simulink model "model"  (R2021a)
settings: Solver=ode45  StartTime=0.0  StopTime=2400  MaxStep=0.1  RelTol=1e-3
values from neighbouring files (symbols this model uses):
  fc_fuel_map_gpkWh = fc_fuel_map./fc_map_kW*3600    [FC_SI95.m]    (also in FC_SI95.mat = [612 612 612 594 558 522 468 522 540 684 756 756 ... (132 el)
  fc_map_spd = [0.5:0.5:6]*1000*2*pi/60    [FC_SI95.m]    (also in FC_SI95.mat = [52.3598775598 104.71975512 157.079632679 209.439510239 261.)
  fc_map_trq = [1:11]*15.6    [FC_SI95.m]    (also in FC_SI95.mat = [15.6 31.2 46.8 62.4 78 93.6 109.2 124.8 140.4 156 171.6])
  mc_eff_map = [0.78 0.79 0.8 0.811 0.811 0.817 0.82 0.828 0.837 0.845 0.862 0.876 ... (1125 elements, 45x25)]    [PM_UQM_motor_100kW.mat]
  mc_map_spd = [0 10.471975512 20.9439510239 31.4159265359 41.8879020479 52.3598775598 62.8318530718 73.3038285838 83.7758040957 94.2477796077 104.71975512 115.191730632 ... (45 elements, 1x45)]    [PM_UQM_motor_100kW.mat]
  mc_map_trq = [-600 -550 -500 -450 -400 -350 -300 -250 -200 -150 -100 -50 ... (25 elements, 1x25)]    [PM_UQM_motor_100kW.mat]
settings Model: Creator=Wlodzimierz  LastModifiedBy=48508
settings SolverCC: ZeroCrossAlgorithm=Adaptive  AlgebraicLoopSolver=TrustRegion
settings DebuggingCC: IgnoredZcDiagnostic=none  SFMachineParentedDataDiag=warning

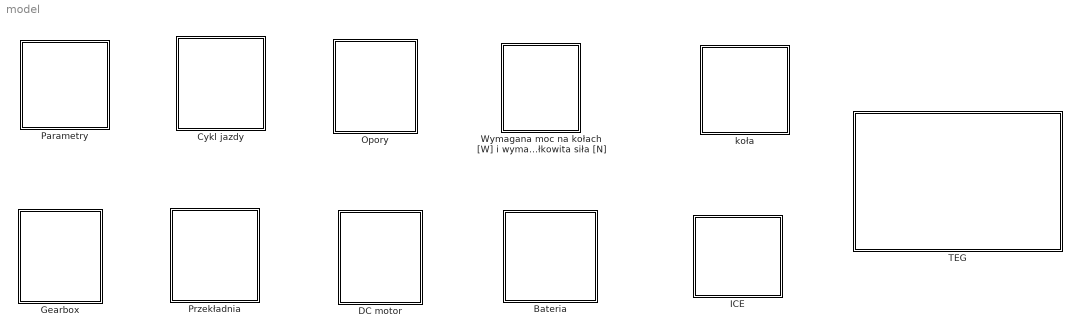
== system model ==
  Bateria : Subsystem
  Cykl jazdy : Subsystem
  DC motor : Subsystem
  Gearbox : Subsystem
  ICE : Subsystem
  Opory : Subsystem
  Parametry : Subsystem  mask{m1_=1500, f1_=0.001, cx_=0.27, a_=2.01, rd_=0.32, prz_=3.46, eta_kwm_=0.95}
      mask prompts: m1_ "masa"; f1_ "wsp. op. tocz."; cx_ "wsp. op. aerodynamicznych cx"; a_ "pow. czołowa [m^2]"; rd_ "promień koła [m]"; prz_ "przełożenie silnik-koła"; eta_kwm_ "sprawność przekładni"
  Przekładnia : Subsystem
  TEG : Subsystem
  Wymagana moc na kołach [W] i wymagana całkowita siła [N] : Subsystem
  koła : Subsystem

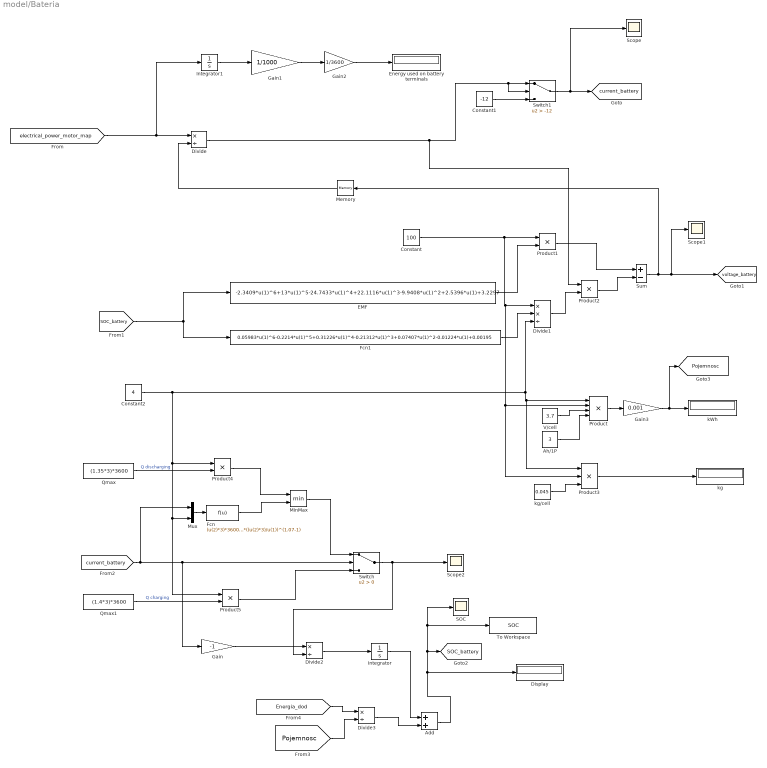
== system model/Bateria ==
  Add : Sum
  Ah/1P : Constant  Value=3
  Constant : Constant  Value=100
  Constant1 : Constant  Value=-12
  Constant2 : Constant  Value=4
  Display : Display
  Divide : Product  Inputs=*/
  Divide1 : Product  Inputs=**/
  Divide2 : Product  Inputs=*/
  Divide3 : Product  Inputs=*/
  EMF : Fcn  Expr=-2.3409*u(1)^6+13*u(1)^5-24.7433*u(1)^4+22.1116*u(1)^3-9.9408*u(1)^2+2.5396*u(1)+3.2297
  Energy used on battery terminals : Display
  Fcn : Fcn  Expr=(u(2)*3)*3600*((u(2)*3)/u(1))^(1.07-1)
  Fcn1 : Fcn  Expr=0.05983*u(1)^6-0.2214*u(1)^5+0.31226*u(1)^4-0.21312*u(1)^3+0.07407*u(1)^2-0.01224*u(1)+0.00195
  Gain : Gain  Gain=-1
  Gain1 : Gain  Gain=1/1000
  Gain2 : Gain  Gain=1/3600
  Gain3 : Gain  Gain=0.001
  Integrator : Integrator  InitialCondition=0.65
  Integrator1 : Integrator
  Memory : Memory  InitialCondition=500
  MinMax : MinMax  Inputs=2  ZeroCross=off
  Mux : Mux  Inputs=2
  Product : Product  Inputs=4
  Product{1..2,4..5} (4 alike) : Product
  Product3 : Product  Inputs=3
  Qmax : Constant  Value=(1.35*3)*3600
  Qmax1 : Constant  Value=(1.4*3)*3600
  SOC : Scope
  Scope : Scope
  Scope1 : Scope
  Scope2 : Scope
  Sum : Sum  Inputs=+-
  Switch : Switch  Criteria=u2 > Threshold  ZeroCross=off
  Switch1 : Switch  Criteria=u2 > Threshold  Threshold=-12
  To Workspace : ToWorkspace  VariableName=SOC  SaveFormat=Timeseries  SampleTime=-1
  V/cell : Constant  Value=3.7
  kWh : Display
  kg : Display
  kg/cell : Constant  Value=0.045
  tag scope: Pojemnosc=global, SOC_battery=global, current_battery=global, voltage_battery=global
  wires:
  Divide/1 -> Product2/1, Switch1/2, Switch1/1
  [SOC_battery] -> EMF/1, Fcn1/1
  Fcn1/1 -> Divide1/2
  Constant2/1 -> Mux/2, Product5/1, Product4/1, Divide1/3, Product3/1, Product/1
  Divide1/1 -> Product2/2
  Product2/1 -> Sum/2
  Sum/1 -> Memory/1, Scope1/1, [voltage_battery]
  EMF/1 -> Product1/2
  Product1/1 -> Sum/1
  Constant/1 -> Product3/2, Product/2, Divide1/1, Product1/1
  Memory/1 -> Divide/2
  Ah/1P/1 -> Product/4
  V/cell/1 -> Product/3
  kg/cell/1 -> Product3/3
  Product3/1 -> kg/1
  Product/1 -> Gain3/1
  Gain/1 -> Divide2/1
  Fcn/1 -> MinMax/2
  MinMax/1 -> Switch/1
  Divide2/1 -> Integrator/1
  Switch/1 -> Scope2/1, Divide2/2
  [current_battery] -> Mux/1, Gain/1, Switch/2
  Qmax/1 -> Product4/2  "Q discharging"
  Mux/1 -> Fcn/1
  Product4/1 -> MinMax/1
  Qmax1/1 -> Product5/2  "Q charging"
  Product5/1 -> Switch/3
  Integrator1/1 -> Gain1/1
  Gain1/1 -> Gain2/1
  Gain2/1 -> Energy used on battery terminals/1
  [electrical_power_motor_map] -> Divide/1, Integrator1/1
  Gain3/1 -> [Pojemnosc], kWh/1
  Constant1/1 -> Switch1/3
  Switch1/1 -> Scope/1, [current_battery]
  [Pojemnosc] -> Divide3/2
  [Energia_dod] -> Divide3/1
  Divide3/1 -> Add/2
  Integrator/1 -> Add/1
  Add/1 -> Display/1, To Workspace/1, SOC/1, [SOC_battery]

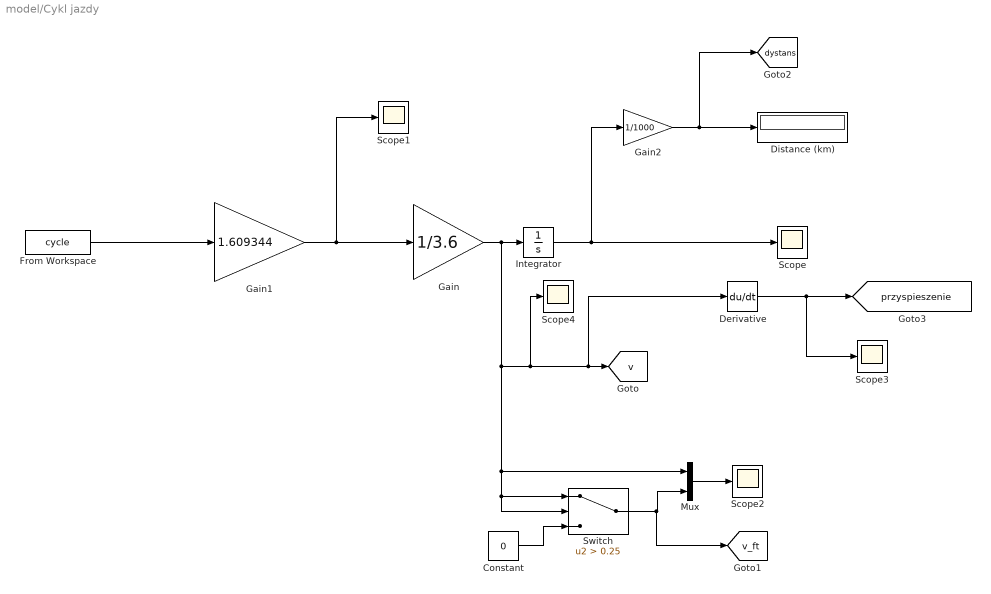
== system model/Cykl jazdy ==
  Constant : Constant  Value=0
  Derivative : Derivative
  Distance (km) : Display
  From Workspace : FromWorkspace  VariableName=cycle
  Gain : Gain  Gain=1/3.6
  Gain1 : Gain  Gain=1.609344
  Gain2 : Gain  Gain=1/1000
  Integrator : Integrator
  Mux : Mux  Inputs=2
  Scope{,1..4} (5 alike) : Scope
  Switch : Switch  Criteria=u2 > Threshold  Threshold=0.25
  tag scope: dystans=global, przyspieszenie=global, v=global, v_ft=global
  wires:
  Mux/1 -> Scope2/1
  Integrator/1 -> Scope/1, Gain2/1
  Gain1/1 -> Gain/1, Scope1/1
  Gain/1 -> Mux/1, Switch/2, Switch/1, Scope4/1, Derivative/1, [v], Integrator/1
  Switch/1 -> [v_ft], Mux/2
  Constant/1 -> Switch/3
  Gain2/1 -> [dystans], Distance (km)/1
  Derivative/1 -> Scope3/1, [przyspieszenie]
  From Workspace/1 -> Gain1/1

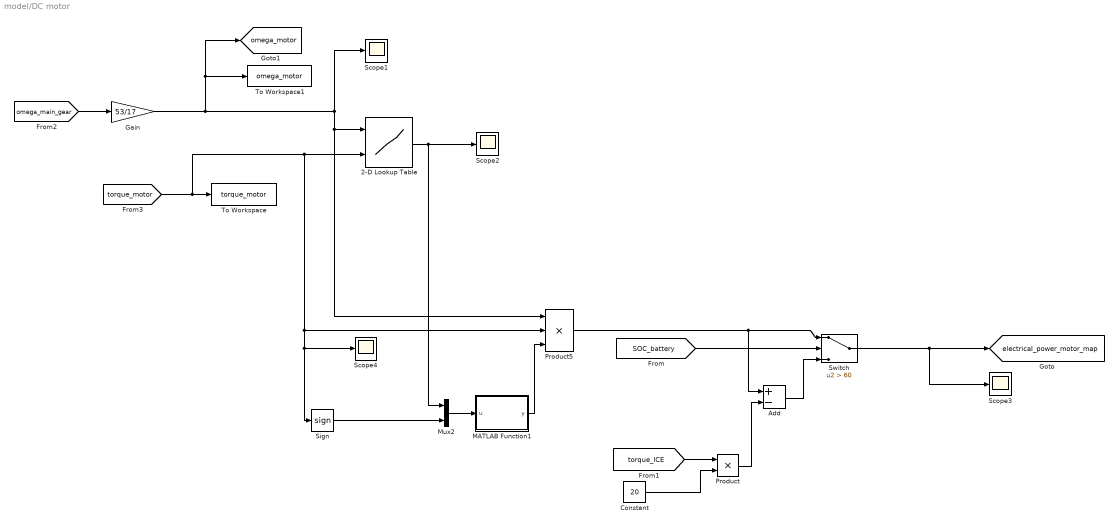
== system model/DC motor ==
  2-D Lookup Table : Lookup_n-D  BreakpointsForDimension1=mc_map_spd*3  BreakpointsForDimension2=mc_map_trq*0.2  Table=mc_eff_map  InternalRulePriority=Speed  RndMeth=Simplest  InputSameDT=on
      settings: InputPortMap=u0,u1
  Add : Sum  Inputs=+-
  Constant : Constant  Value=20
  Gain : Gain  Gain=53/17
  MATLAB Function1 : MATLAB Function  TreatAsAtomicUnit=on
  Mux2 : Mux  Inputs=2
  Product : Product
  Product5 : Product  Inputs=3
  Scope{1..4} (4 alike) : Scope
  Sign : Signum
  Switch : Switch  Criteria=u2 > Threshold  Threshold=60
  To Workspace : ToWorkspace  VariableName=torque_motor  SampleTime=1
  To Workspace1 : ToWorkspace  VariableName=omega_motor  SampleTime=1
  tag scope: electrical_power_motor_map=global, omega_motor=global
  wires:
  Sign/1 -> Mux2/2
  2-D Lookup Table/1 -> Mux2/1, Scope2/1
  Mux2/1 -> MATLAB Function1/1(u)
  MATLAB Function1/1(y) -> Product5/3
  [torque_motor] -> Scope4/1, Sign/1, Product5/2, 2-D Lookup Table/2, To Workspace/1
  [omega_main_gear] -> Gain/1
  [torque_ICE] -> Product/1
  Constant/1 -> Product/2
  [SOC_battery] -> Switch/2
  Product5/1 -> Add/1, Switch/1
  Product/1 -> Add/2
  Add/1 -> Switch/3
  Switch/1 -> Scope3/1, [electrical_power_motor_map]
  Gain/1 -> [omega_motor], To Workspace1/1, Product5/1, 2-D Lookup Table/1, Scope1/1

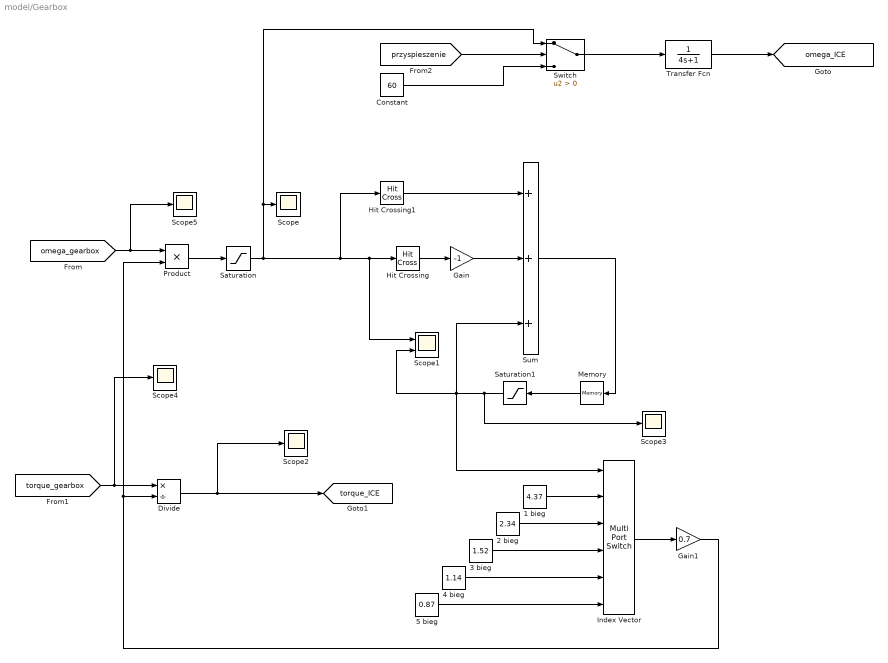
== system model/Gearbox ==
  1 bieg : Constant  Value=4.37
  2 bieg : Constant  Value=2.34
  3 bieg : Constant  Value=1.52
  4 bieg : Constant  Value=1.14
  5 bieg : Constant  Value=0.87
  Constant : Constant  Value=60
  Divide : Product  Inputs=*/
  Gain : Gain  Gain=-1
  Gain1 : Gain  Gain=0.7
  Hit Crossing : HitCross  HitCrossingOffset=120  HitCrossingDirection=falling
  Hit Crossing1 : HitCross  HitCrossingOffset=270  HitCrossingDirection=rising
  Index Vector : MultiPortSwitch  Inputs=5
  Memory : Memory  InitialCondition=1
  Product : Product
  Saturation : Saturate  UpperLimit=280  LowerLimit=80
  Saturation1 : Saturate  UpperLimit=5  LowerLimit=1
  Scope{,2..5} (5 alike) : Scope
  Scope1 : Scope  NumInputPorts=2
  Sum : Sum  Inputs=+++
  Switch : Switch  Criteria=u2 > Threshold
  Transfer Fcn : TransferFcn  Denominator=[4 1]
  tag scope: omega_ICE=global, torque_ICE=global
  wires:
  [omega_gearbox] -> Scope5/1, Product/1
  Product/1 -> Saturation/1
  Saturation/1 -> Switch/1, Scope/1, Scope1/1, Hit Crossing/1, Hit Crossing1/1
  Hit Crossing/1 -> Gain/1
  Hit Crossing1/1 -> Sum/1
  Gain/1 -> Sum/2
  Sum/1 -> Memory/1
  Memory/1 -> Saturation1/1
  Saturation1/1 -> Scope3/1, Index Vector/1, Scope1/2, Sum/3
  [torque_gearbox] -> Scope4/1, Divide/1
  Gain1/1 -> Product/2, Divide/2
  5 bieg/1 -> Index Vector/6
  4 bieg/1 -> Index Vector/5
  3 bieg/1 -> Index Vector/4
  2 bieg/1 -> Index Vector/3
  1 bieg/1 -> Index Vector/2
  Index Vector/1 -> Gain1/1
  Divide/1 -> Scope2/1, [torque_ICE]
  [przyspieszenie] -> Switch/2
  Constant/1 -> Switch/3
  Switch/1 -> Transfer Fcn/1
  Transfer Fcn/1 -> [omega_ICE]

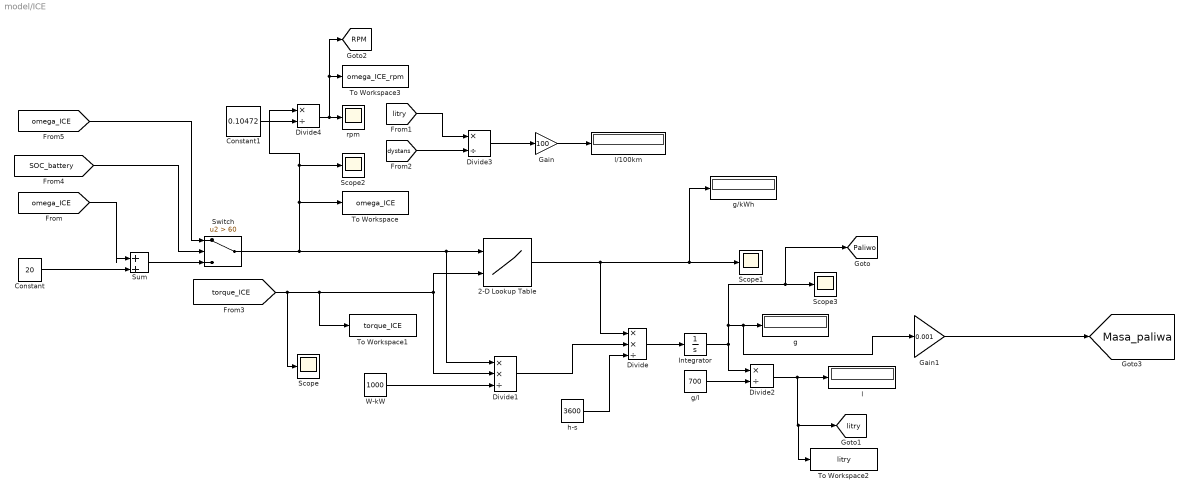
== system model/ICE ==
  2-D Lookup Table : Lookup_n-D  BreakpointsForDimension1=fc_map_spd  BreakpointsForDimension2=fc_map_trq  Table=fc_fuel_map_gpkWh  InternalRulePriority=Speed  RndMeth=Simplest  InputSameDT=on
      settings: InputPortMap=u0,u1
  Constant : Constant  Value=20
  Constant1 : Constant  Value=0.10472
  Divide : Product  Inputs=**/
  Divide1 : Product  Inputs=**/
  Divide2 : Product  Inputs=*/
  Divide3 : Product  Inputs=*/
  Divide4 : Product  Inputs=*/
  Gain : Gain  Gain=100
  Gain1 : Gain  Gain=0.001
  Integrator : Integrator
  Scope{,1..3} (4 alike) : Scope
  Sum : Sum  Inputs=|++
  Switch : Switch  Criteria=u2 > Threshold  Threshold=60
  To Workspace : ToWorkspace  VariableName=omega_ICE  SampleTime=1
  To Workspace1 : ToWorkspace  VariableName=torque_ICE  SampleTime=1
  To Workspace2 : ToWorkspace  VariableName=litry  SaveFormat=Timeseries  SampleTime=-1
  To Workspace3 : ToWorkspace  VariableName=omega_ICE_rpm  SampleTime=1
  W-kW : Constant  Value=1000
  g : Display
  g/kWh : Display
  g/l : Constant  Value=700
  h-s : Constant  Value=3600
  l : Display
  l/100km : Display
  rpm : Scope
  tag scope: Masa_paliwa=global, Paliwo=global, RPM=global, litry=global
  wires:
  W-kW/1 -> Divide1/3
  Divide1/1 -> Divide/2
  Divide/1 -> Integrator/1
  h-s/1 -> Divide/3
  g/l/1 -> Divide2/2
  Integrator/1 -> Gain1/1, g/1, [Paliwo], Scope3/1, Divide2/1
  Divide2/1 -> To Workspace2/1, [litry], l/1
  2-D Lookup Table/1 -> g/kWh/1, Scope1/1, Divide/1
  [dystans] -> Divide3/2
  [litry] -> Divide3/1
  Divide3/1 -> Gain/1
  Gain/1 -> l/100km/1
  [torque_ICE] -> Scope/1, To Workspace1/1, Divide1/2, 2-D Lookup Table/2
  [omega_ICE] -> Sum/1
  Constant/1 -> Sum/2
  [SOC_battery] -> Switch/2
  Sum/1 -> Switch/3
  Switch/1 -> Divide4/1, Scope2/1, To Workspace/1, Divide1/1, 2-D Lookup Table/1
  [omega_ICE] -> Switch/1
  Constant1/1 -> Divide4/2
  Divide4/1 -> [RPM], To Workspace3/1, rpm/1
  Gain1/1 -> [Masa_paliwa]

== system model/Opory ==
  sila oporow bezwladnosci [N] : Subsystem
  sila oporów toczenia [N] : Subsystem
  siła oporów aerodynamicznych [N] : Subsystem

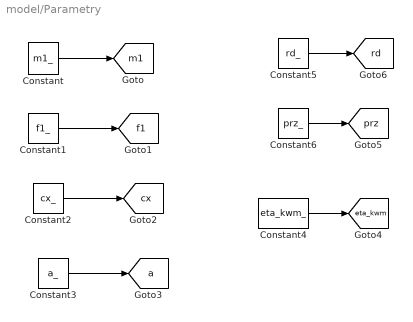
== system model/Parametry ==
  Constant : Constant  Value=m1_
  Constant1 : Constant  Value=f1_
  Constant2 : Constant  Value=cx_
  Constant3 : Constant  Value=a_
  Constant4 : Constant  Value=eta_kwm_
  Constant5 : Constant  Value=rd_
  Constant6 : Constant  Value=prz_
  tag scope: a=global, cx=global, eta_kwm=global, f1=global, m1=global, prz=global, rd=global
  wires:
  Constant1/1 -> [f1]
  Constant/1 -> [m1]
  Constant5/1 -> [rd]
  Constant2/1 -> [cx]
  Constant3/1 -> [a]
  Constant4/1 -> [eta_kwm]
  Constant6/1 -> [prz]

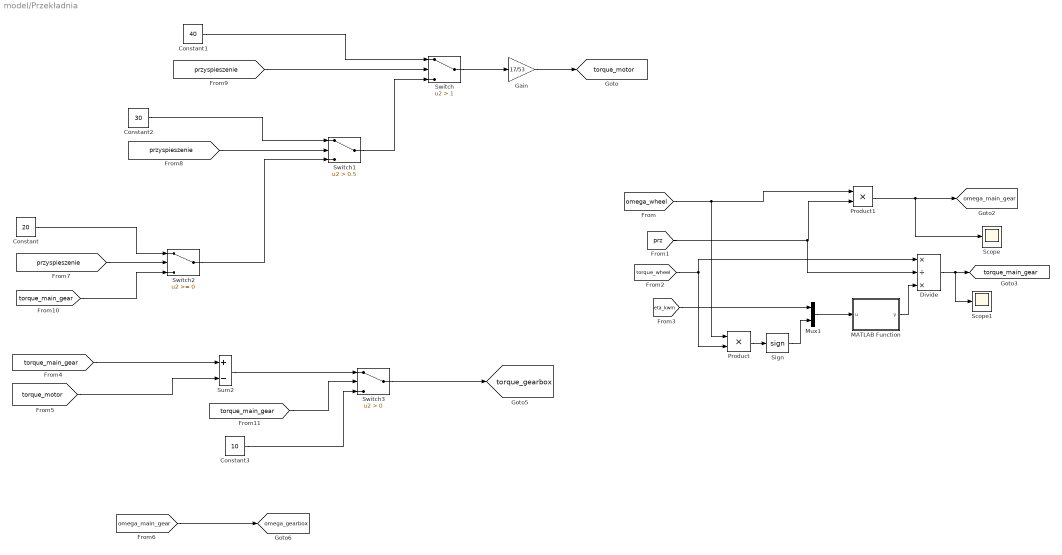
== system model/Przekładnia ==
  Constant : Constant  Value=20
  Constant1 : Constant  Value=40
  Constant2 : Constant  Value=30
  Constant3 : Constant  Value=10
  Divide : Product  Inputs=*/*
  Gain : Gain  Gain=17/53
  MATLAB Function : MATLAB Function  TreatAsAtomicUnit=on
  Mux1 : Mux  Inputs=2
  Product : Product
  Product1 : Product
  Scope : Scope
  Scope1 : Scope
  Sign : Signum
  Sum2 : Sum  Inputs=+-
  Switch : Switch  Criteria=u2 > Threshold  Threshold=1
  Switch1 : Switch  Criteria=u2 > Threshold  Threshold=0.5
  Switch2 : Switch
  Switch3 : Switch  Criteria=u2 > Threshold
  tag scope: omega_gearbox=global, omega_main_gear=global, torque_gearbox=global, torque_main_gear=global, torque_motor=global
  wires:
  MATLAB Function/1(y) -> Divide/3
  Product/1 -> Sign/1
  Divide/1 -> Scope1/1, [torque_main_gear]
  [torque_wheel] -> Product/2, Divide/1
  [eta_kwm] -> Mux1/1
  [omega_wheel] -> Product/1, Product1/1
  Mux1/1 -> MATLAB Function/1(u)
  [prz] -> Divide/2, Product1/2
  Product1/1 -> Scope/1, [omega_main_gear]
  Sign/1 -> Mux1/2
  [torque_main_gear] -> Sum2/1
  [torque_motor] -> Sum2/2
  [przyspieszenie] -> Switch2/2
  [torque_main_gear] -> Switch2/3
  Constant/1 -> Switch2/1
  Switch2/1 -> Switch1/3
  [przyspieszenie] -> Switch1/2
  Switch1/1 -> Switch/3
  [przyspieszenie] -> Switch/2
  Constant2/1 -> Switch1/1
  Constant1/1 -> Switch/1
  Switch/1 -> Gain/1
  Gain/1 -> [torque_motor]
  [omega_main_gear] -> [omega_gearbox]
  Switch3/1 -> [torque_gearbox]
  Sum2/1 -> Switch3/1
  [torque_main_gear] -> Switch3/2
  Constant3/1 -> Switch3/3

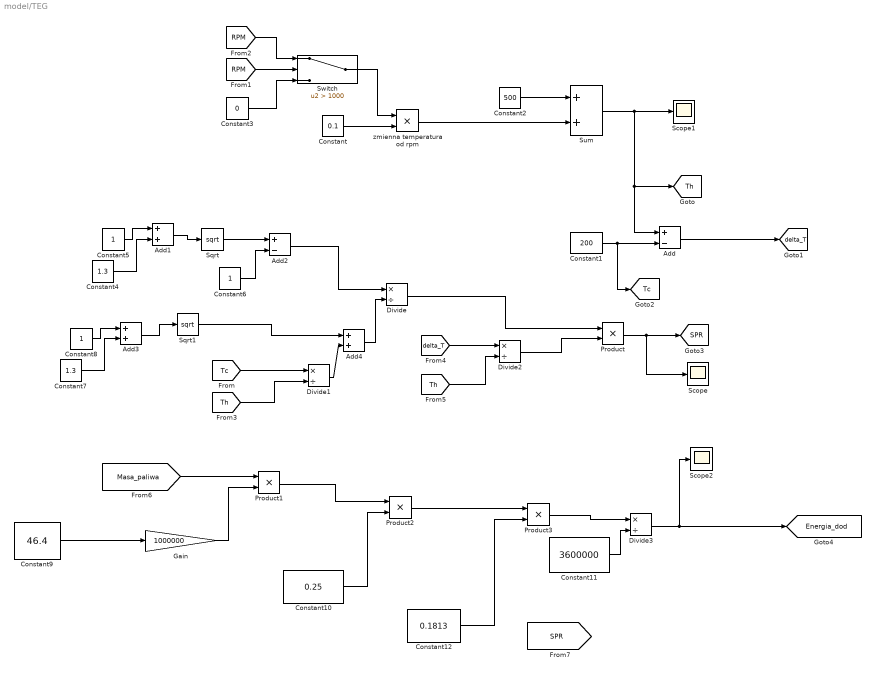
== system model/TEG ==
  Add : Sum  Inputs=+-
  Add1 : Sum
  Add2 : Sum  Inputs=+-
  Add3 : Sum
  Add4 : Sum
  Constant : Constant  Value=0.1
  Constant1 : Constant  Value=200
  Constant10 : Constant  Value=0.25
  Constant11 : Constant  Value=3600000
  Constant12 : Constant  Value=0.1813
  Constant2 : Constant  Value=500
  Constant3 : Constant  Value=0
  Constant4 : Constant  Value=1.3
  Constant5 : Constant
  Constant6 : Constant
  Constant7 : Constant  Value=1.3
  Constant8 : Constant
  Constant9 : Constant  Value=46.4
  Divide{,1..3} (4 alike) : Product  Inputs=*/
  Gain : Gain  Gain=1000000
  Product{,1..3} (4 alike) : Product
  Scope : Scope
  Scope1 : Scope
  Scope2 : Scope
  Sqrt : Sqrt  SaturateOnIntegerOverflow=on
  Sqrt1 : Sqrt  SaturateOnIntegerOverflow=on
  Sum : Sum
  Switch : Switch  Criteria=u2 > Threshold  Threshold=1000
  zmienna temperatura od rpm : Product  Inputs=**
  tag scope: Energia_dod=global, SPR=global, Tc=global, Th=global, delta_T=global
  wires:
  Constant/1 -> zmienna temperatura od rpm/2
  Constant2/1 -> Sum/1
  Sum/1 -> [Th], Add/1, Scope1/1
  zmienna temperatura od rpm/1 -> Sum/2
  [RPM] -> Switch/2
  Constant3/1 -> Switch/3
  Switch/1 -> zmienna temperatura od rpm/1
  [RPM] -> Switch/1
  Constant1/1 -> [Tc], Add/2
  Add/1 -> [delta_T]
  Constant5/1 -> Add1/1
  Constant4/1 -> Add1/2
  Add1/1 -> Sqrt/1
  Sqrt/1 -> Add2/1
  Constant6/1 -> Add2/2
  Add2/1 -> Divide/1
  Constant7/1 -> Add3/2
  Constant8/1 -> Add3/1
  Add3/1 -> Sqrt1/1
  [Tc] -> Divide1/1
  [Th] -> Divide1/2
  Sqrt1/1 -> Add4/1
  Divide1/1 -> Add4/2
  Add4/1 -> Divide/2
  [delta_T] -> Divide2/1
  [Th] -> Divide2/2
  Divide/1 -> Product/1
  Divide2/1 -> Product/2
  Product/1 -> Scope/1, [SPR]
  Constant9/1 -> Gain/1
  Gain/1 -> Product1/2
  [Masa_paliwa] -> Product1/1
  Product1/1 -> Product2/1
  Constant10/1 -> Product2/2
  Product2/1 -> Product3/1
  Product3/1 -> Divide3/1
  Constant11/1 -> Divide3/2
  Divide3/1 -> [Energia_dod], Scope2/1
  Constant12/1 -> Product3/2

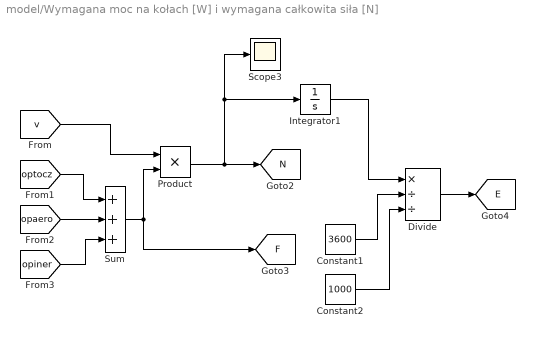
== system model/Wymagana moc na kołach [W] i wymagana całkowita siła [N] ==
  Constant1 : Constant  Value=3600
  Constant2 : Constant  Value=1000
  Divide : Product  Inputs=*//
  Integrator1 : Integrator
  Product : Product
  Scope3 : Scope
  Sum : Sum  Inputs=+++
  tag scope: E=global, F=global, N=global
  wires:
  [opiner] -> Sum/3
  Constant1/1 -> Divide/2
  Constant2/1 -> Divide/3
  [optocz] -> Sum/1
  Divide/1 -> [E]
  [opaero] -> Sum/2
  Product/1 -> Scope3/1, Integrator1/1, [N]
  Integrator1/1 -> Divide/1
  Sum/1 -> Product/2, [F]
  [v] -> Product/1

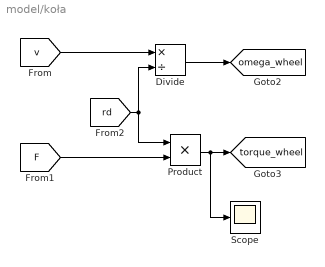
== system model/koła ==
  Divide : Product  Inputs=*/
  Product : Product
  Scope : Scope
  tag scope: omega_wheel=global, torque_wheel=global
  wires:
  [rd] -> Product/1, Divide/2
  Product/1 -> Scope/1, [torque_wheel]
  [F] -> Product/2
  [v] -> Divide/1
  Divide/1 -> [omega_wheel]

== system model/Opory/sila oporow bezwladnosci [N] ==
  Derivative : Derivative
  Product : Product
  Przyspieszenie : Scope
  tag scope: opiner=global
  wires:
  [v] -> Derivative/1
  Derivative/1 -> Przyspieszenie/1, Product/1
  [m1] -> Product/2
  Product/1 -> [opiner]

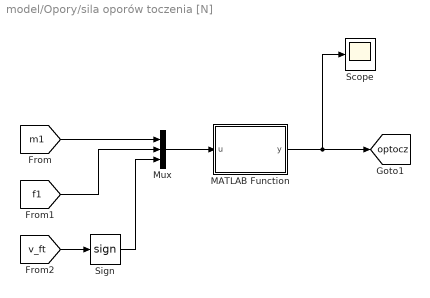
== system model/Opory/sila oporów toczenia [N] ==
  MATLAB Function : MATLAB Function  TreatAsAtomicUnit=on
  Mux : Mux  Inputs=3
  Scope : Scope
  Sign : Signum
  tag scope: optocz=global
  wires:
  [f1] -> Mux/2
  Mux/1 -> MATLAB Function/1(u)
  [m1] -> Mux/1
  [v_ft] -> Sign/1
  Sign/1 -> Mux/3
  MATLAB Function/1(y) -> Scope/1, [optocz]

== system model/Opory/siła oporów aerodynamicznych [N] ==
  MATLAB Function : MATLAB Function  TreatAsAtomicUnit=on
  Mux1 : Mux  Inputs=3
  Scope : Scope
  tag scope: opaero=global
  wires:
  [v] -> Mux1/3
  Mux1/1 -> MATLAB Function/1(u)
  MATLAB Function/1(y) -> Scope/1, [opaero]
  [a] -> Mux1/2
  [cx] -> Mux1/1

== matlab function model/Opory/sila oporów toczenia [N]/MATLAB Function ==
  data: u input; y output
function y = fcn(u)

y = u(1)*9.81*u(2)*u(3);

== matlab function model/Przekładnia/MATLAB Function ==
  data: u input; y output
function y = fcn(u)

y = u(1)^(-u(2));

== matlab function model/DC motor/MATLAB Function1 ==
  data: u input; y output
function y = fcn(u)

y = u(1)^(-u(2));

== matlab function model/Opory/siła oporów aerodynamicznych [N]/MATLAB Function ==
  data: u input; y output
function y = fcn(u)


y = 0.5*1.23*u(1)*u(2)*u(3)*u(3);
